simulink model "Controller_Template"  (R2020a)
settings: Solver=FixedStepAuto  StartTime=0.0  StopTime=TMax  FixedStep=DT  RelTol=1e-3  EnableMultiTasking=on
settings Model: Creator=lpwoolcock  LastModifiedBy=lpwoolcock

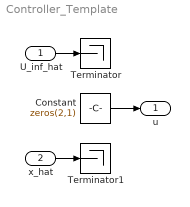
== system Controller_Template ==
  U_inf_hat : Inport  PortDimensions=1
  x_hat : Inport  Port=2  PortDimensions=[5 1]
  Constant : Constant  Value=zeros(2,1)
  Terminator : Terminator
  Terminator1 : Terminator
  u : Outport  PortDimensions=[2 1]
  wires:
  Constant/1 -> u/1
  U_inf_hat/1 -> Terminator/1
  x_hat/1 -> Terminator1/1
